simulink model "RedCrane_Merged_control_12032025"  (R2024b)
settings: Solver=VariableStepAuto  StartTime=0.0  StopTime=33  RelTol=1e-4
model workspace (MATLAB code in the model file):
  | %% Geometric properties
  | 
  | %Basic geometry width
  | w0 = 0.07;
  | w1 = w0/4;
  | l_RJ = 0.277; %2.1*w0;
  | r_RJ = 0.030;
  | 
  | %Column geometry
  | L_Column = 1.5655; %2;
  | eta_B = -0.25;
  | zeta_B = L_Column;
  | eta_D = -0.365; %0.25;
  | zeta_D = 1.4805; %1.5;
  | eta_J = 0.200; % 0.25;
  | zeta_J = 0.1195; %0.25;
  | 
  | %Column - Main boom link
  | l_DE = 0.490; % 0.5;
  | l_FE = 0.170; % 0.4;
  | 
  | %Main boom geometry
  | L_Mboom = 2.400; % 2;
  | eta_C = 2.400; % 2;
  | zeta_C = 0.070; % 0.25;
  | eta_F = 0.340; % 0.6;
  | zeta_F = 0.010; % -0.25;
  | eta_G = 2.365; % 1.75;
  | zeta_G = 0.235; % -0.25;
  | eta_K = 0.750; % 1;
  | zeta_K = 0.045; % -0.25;
  | 
  | %Main boom-Jib boom link
  | l_GH = 0.490; % 0.5;
  | l_IH = 0.220; % 0.4;
  | 
  | %Jib boom geometry
  | L_Jib_boom = 2.429; % 2;
  | eta_I = 0.280; % 0.5;
  | zeta_I = 0.005; % -0.25;
  | eta_TP = L_Jib_boom;
  | zeta_TP = 0;
  | 
  | % Winch
  | r_W = 0.205/2;
  | L_W = 0.191;
  | eta_W = 0.28722;
  | zeta_W = -0.29926;
  | beta_W = -0.335;
  | 
  | % Mounting plate
  | eta_MP = -0.0249;
  | zeta_MP = -0.17479;
  | beta_MP = 0;
  | 
  | % Pulley
  | r_P = 0.210/2; % Radius pulley
  | eta_P = 2.140;
  | zeta_P = -0.0506;
  | beta_P = -0.0;
  | 
  | %Roller
  | r_RO = 0.055/2; % Radius roller over
  | r_RU = 0.046/2; % Radius roller under
  | eta_RO = 0.306;
  | zeta_RO = 0.12510;
  | 
  | %Mounting
  | L_M = 1; %m
  | W_M = 1; %m
  | H_M = 1; %m
  | eta_M = 0; %m
  | zeta_M = -0.5; %m
  | beta_M = 0; %m
  | 
  | %Ground
  | L_ground = 6; %m
  | W_ground = 4; %m
  | H_ground = 0.01; %m
  | eta_ground = 1.5; %m
  | zeta_ground = -0.5; %m
  | beta_ground = 0; %m
  | 
  | 
  | %% Mass properties (Mass and center of mass)
  | column_mass = 239.4; % kg
  | column_COM = [-0.1007, 0.0001, 0.4351]; % m
  | 
  | MainBoom_mass = 216.5; % kg
  | MainBoom_COM = [1.134, 0.1674, -0.0018]; % m
  | 
  | JibBoom_mass = 842.2; % kg
  | JibBoom_COM = [0.9806, 0.1814, -0.2939]; % m
  | 
  | % Dogbone
  | E2F_mass = 7.076*2; % kg
  | E2F_COM = [0.0817, 0, 0]; % m
  | 
  | D2E_mass = 6.426*2; % kg
  | D2E_COM = [0.245, 0, 0]; % m
  | 
  | G2H_mass = 6.426*2; % kg
  | G2H_COM = [0.245, 0, 0]; % m
  | 
  | H2I_mass = 22.05; % kg
  | H2I_COM = [0.1206, 0, 0]; % m
  | 
  | % Main cylinder
  | MainC_bottom_mass = 57.9561; % kg
  | MainC_bottom_COM = [0.0081, -0.001, 0.4125]; % m
  | 
  | MainC_rod_mass = 43.93; % kg
  | MainC_rod_COM = [0, 0, -0.4290]; % m
  | 
  | % Jib cylinder
  | JibC_bottom_mass = 55.7738; % kg
  | JibC_bottom_COM = [0.0038, 0.0022, 0.4468]; % m
  | 
  | JibC_rod_mass = 45.8854; % kg
  | JibC_rod_COM = [0, 0, -0.4694]; % m
  | 
  | % Winch
  | Winch_mass = 54; % kg
  | Winch_COM = [0, 0, 0]; % m
  | 
  | 
  | %% Inertia properties (Moments of inertia and products of inertia)
  | 
  | column_MOI = [109, 114, 9.009]; % kg*m^2
  | column_POI = [0.0319, -21.59, -0.0113]; % kg*m^2
  | 
  | MainBoom_MOI = [6.5, 160.3, 160]; % kg*m^2
  | MainBoom_POI = [0.0666, 0.1093, 8.016]; % kg*m^2
  | 
  | JibBoom_MOI = [31.75, 566.3, 573.1]; % kg*m^2
  | JibBoom_POI = [-0.0237, -11.42, 9.588]; % kg*m^2
  | 
  | % Dogbone
  | E2F_MOI = [0.0111, 0.0546, 0.0587]; % kg*m^2
  | E2F_POI = [0, -0.0089, 0]; % kg*m^2
  | 
  | D2E_MOI = [0.0069, 0.2419, 0.2485]; % kg*m^2
  | D2E_POI = [0, 0, 0]; % kg*m^2
  | 
  | G2H_MOI = [0.0069, 0.2419, 0.2485]; % kg*m^2
  | G2H_POI = [0, 0, 0]; % kg*m^2
  | 
  | H2I_MOI = [0.2636, 0.4184, 0.1901]; % kg*m^2
  | H2I_POI = [0, 0, 0]; % kg*m^2
  | 
  | 
  | % Main cylinder
  | MainC_bottom_MOI = [7.2059, 7.2304, 0.3979]; % kg*m^2
  | MainC_bottom_POI = [-0.0126, -0.1802, 0.0002]; % kg*m^2
  | 
  | MainC_rod_MOI = [6.0014, 5.9633, 0.1401]; % kg*m^2
  | MainC_rod_POI = [0, -0.0001, 0]; % kg*m^2
  | 
  | % Jib cylinder
  | JibC_bottom_MOI = [8.3780, 8.3476, 0.3607]; % kg*m^2
  | JibC_bottom_POI = [-0.0119, -0.1037, 0.0033]; % kg*m^2
  | 
  | JibC_rod_MOI = [7.4245, 7.3864, 0.1401]; % kg*m^2
  | JibC_rod_POI = [0, -0.0001, 0]; % kg*m^2
  | 
  | % Winch
  | I_W_xx = (1/4)*Winch_mass*r_W^2 + (1/12)*Winch_mass*L_W^2;
  | I_W_yy = (1/4)*Winch_mass*r_W^2 + (1/12)*Winch_mass*L_W^2;
  | I_W_zz = (1/2)*Winch_mass*r_W^2;
  | 
  | Winch_MOI = [I_W_xx, I_W_yy, I_W_zz]; % kg*m^2
  | Winch_POI = [0, 0, 0]; % kg*m^2
  | 
  | 
  | %% Hydraulics
  | 
  | %-------------Cylinder---------------------
  | 
  | % Main cylinder
  | D_piston_MainC = 160; %mm dimater of piston side
  | L_piston_MainC = 65; %66.2;%mm length from joint to buttom of piston side
  | D_rod_MainC = 100; %mm diamter of cylinder rod
  | L_rod_MainC = 978; %990;%mm length from bottom of rod to joint
  | A_piston_MainC = pi/4*D_piston_MainC^2; % mm^2 area of piston side
  | A_rod_MainC = pi/4*D_rod_MainC^2; % mm^2 area of rod
  | A_rodside_MainC = A_piston_MainC-A_rod_MainC; % mm^2 area of rod side
  | L_barrel_MainC = 945-L_piston_MainC; %mm
  | stroke_MainC = 0.75; %m
  | initial_pos_Main = 0.18; %m
  | initial_Pa_Main = 17;%Bar
  | 
  | % Jib cylinder
  | D_piston_JibC = 150; %mm dimater of piston side
  | L_piston_JibC = 65; %66.2;%mm length from joint to buttom of piston side
  | D_rod_JibC = 100; %mm diamter of cylinder rod
  | L_rod_JibC = 1089.5; %1105.5;%mm length from bottom of rod to joint
  | A_piston_JibC = pi/4*D_piston_JibC^2; % mm^2 area of piston side
  | A_rod_JibC = pi/4*D_rod_JibC^2; % mm^2 area of rod
  | A_rodside_JibC = A_piston_JibC-A_rod_JibC; % mm^2 area of rod side
  | L_barrel_JibC = 1050-L_piston_JibC; %mm
  | stroke_JibC = 0.855; %m
  | initial_pos_Jib = 0.855; %m
  | initial_Pa_Jib = 1;%Bar
  | initial_Pb_Jib = 67;%Bar
  | 
  | % winch
  | poly_b = [1.762740809095876e+02,-44.442169999547330];
  | poly_c = [1.901177983521692e+02,-1.484122102902541e+02];
  | angle_b = poly_b(1)*initial_pos_Main + poly_b(2);
  | angle_c = poly_c(1)*initial_pos_Jib + poly_c(2);
  | angle_w = -90 - angle_c - angle_b;
  | 
  | %Motor
  | DM = 200; %Displacement cm^3/rev
  | GR = 5.04; % Gear ratio 1:5,04
  | 
  | 
  | % ------------------CBV-------------------
  | 
  | % Main
  | pCr_Main = 43.95;%Bar
  | dp_open_Main = 124.43;%Bar
  | 
  | % Jib
  | alpha = 2.7;
  | pCr_Jib_A = 320;%Bar
  | dp_open_Jib_A = 65;%Bar
  | pCr_Jib_B = 280;%Bar
  | dp_open_Jib_B = 40;%Bar
  | 
  | %-------------------DCV-----------------------
  | Cd = 0.64;
  | Q_rat = 30/6e4;
  | dp_2 = 6e5;
  | dp_1 = 1e5;
  | roh = 850;
  | 
  | % Main dcv
  | dead_up_Main = 0.071;
  | dead_down_Main = 0.126;
  | 
  | % Jib dcv
  | dead_up_Jib = 0.037;
  | dead_down_Jib = 0.126;
  | 
  | Ad2 = Q_rat/(Cd*sqrt(2/roh*dp_2))*1e6; %mm
  | Ad1_1 = Q_rat/(Cd*sqrt(2/roh*dp_1))*1e6;
  | Ad1_0 = Q_rat/(Cd*sqrt(2/roh*dp_1))*1e6*0;
  | 
  | Ad1_Main_up = Q_rat/(Cd*sqrt(2/roh*dp_1))*1e6*dead_up_Main;
  | Ad1_Main_down = Q_rat/(Cd*sqrt(2/roh*dp_1))*1e6*dead_down_Main;
  | Ad1_Jib_up = Q_rat/(Cd*sqrt(2/roh*dp_1))*1e6*dead_up_Jib;
  | Ad1_Jib_down = Q_rat/(Cd*sqrt(2/roh*dp_1))*1e6*dead_down_Jib;
undefined symbols (not defined in the file or in its folder): dead_down_m, dead_up_m, X, Y, Z
libraries: sm_lib x171, fl_lib x94, nesl_utility x64, SimscapeFluids_lib x33, sdl_lib x1
(part 4 of 9)

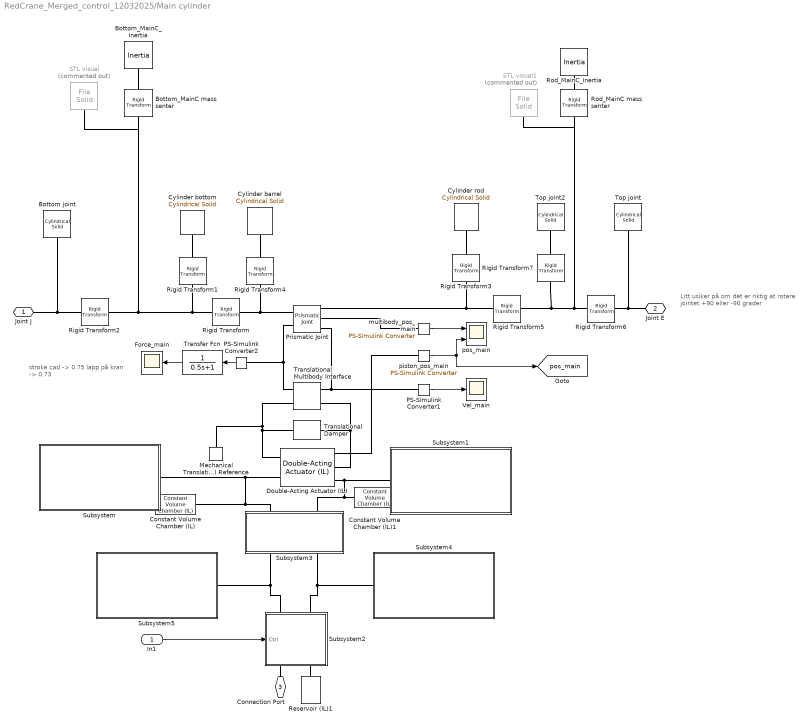
== system RedCrane_Merged_control_12032025/Main cylinder ==
  note: stroke
      | cad -> 0.75
      | lapp på kran -> 0.73
  note: Litt usiker på om det er riktig
      | at rotere jointet +90 eller -90
      | grader
  In1 : Inport
  Bottom joint : sm_lib/Body Elements/Cylindrical Solid  CylinderRadius=0.05  CylinderRadiusUnits=m  CylinderLength=0.2  CylinderLengthUnits=m  ExportEntireGeometry=off  InertiaType=Custom  BasedOnType=Density  Density=1000  DensityUnits=kg/m^3  Mass=0  MassUnits=kg  CenterOfMass=[0 0 0]  CenterOfMassUnits=m  MomentsOfInertia=[0 0 0]  MomentsOfInertiaUnits=kg*m^2  ProductsOfInertia=[0 0 0]  ProductsOfInertiaUnits=kg*m^2  GraphicType=FromGeometry  MarkerShape=Sphere  MarkerSize=10  GraphicVisPropType=SimpleVisualProperties  GraphicDiffuseColor=[0 1 0]  GraphicOpacity=1  GraphicSpecularColor=[0.5 0.5 0.5 1.0]  GraphicAmbientColor=[0.15 0.15 0.15 1.0]  GraphicEmissiveColor=[0.0 0.0 0.0 1.0]  GraphicShininess=75  DoExposeReferenceFrame=on  SerializedFrames=<Frames/>
  Bottom_MainC mass senter : sm_lib/Frames and Transforms/Rigid Transform  RotationMethod=None  FollAlignAxisA=+X  BaseAlignAxisA=+Y  FollAlignAxisB=+Y  BaseAlignAxisB=+Z  RotationStandardAxis=+Z  RotationAngle=0  RotationAngleUnits=deg  RotationArbitraryAxis=[0 0 1]  RotationSequenceAxes=FollowerAxes  RotationSequence=XYX  RotationSequenceAngles=[0 0 0]  RotationSequenceAnglesUnits=deg  RotationMatrix=[1 0 0;0 1 0;0 0 1]  Quaternion=[1 0 0 0]  TranslationMethod=Cartesian  TranslationCartesianOffset=MainC_bottom_COM  TranslationCartesianOffsetUnits=m  TranslationStandardAxis=+Z  TranslationStandardOffset=0  TranslationStandardOffsetUnits=m  TranslationROffset=0  TranslationROffsetUnits=m  TranslationThetaOffset=0  TranslationThetaOffsetUnits=deg  TranslationZOffset=0  TranslationZOffsetUnits=m
  Bottom_MainC_Inertia : sm_lib/Body Elements/Inertia  InertiaType=Custom  Mass=MainC_bottom_mass  MassUnits=kg  CenterOfMass=[0,0,0]  CenterOfMassUnits=m  MomentsOfInertia=MainC_bottom_MOI  MomentsOfInertiaUnits=kg*m^2  ProductsOfInertia=MainC_bottom_POI  ProductsOfInertiaUnits=kg*m^2  GraphicType=Marker  MarkerShape=Sphere  MarkerSize=20  GraphicVisPropType=SimpleVisualProperties  GraphicDiffuseColor=[1 0 1]  GraphicOpacity=1  GraphicSpecularColor=[0.5 0.5 0.5 1.0]  GraphicAmbientColor=[0.15 0.15 0.15 1.0]  GraphicEmissiveColor=[0.0 0.0 0.0 1.0]  GraphicShininess=75
  Constant Volume Chamber (IL) : fl_lib/Isothermal Liquid/Elements/Constant Volume Chamber (IL)  volume=0.001 m^3  p_I_specify=on  p_I_priority=High  p_I=initial_Pa_Main bar  p_I_nominal_specify=off  p_I_nominal_value=1  p_I_nominal_unit=MPa
      settings: InternalSimscapePortConfiguration="{\"Bottom\":[],\"Left\":[{\"id\":\"A\",\"label\":\"A\",\"type\":\"foundation.isothermal_liquid.isothermal_liquid\"}],\"Right\":[],\"Top\":[]}"
  Constant Volume Chamber (IL)1 : fl_lib/Isothermal Liquid/Elements/Constant Volume Chamber (IL)  volume=0.001 m^3  p_I_specify=on  p_I_priority=High  p_I=47 bar  p_I_nominal_specify=off  p_I_nominal_value=1  p_I_nominal_unit=MPa
      settings: InternalSimscapePortConfiguration="{\"Bottom\":[],\"Left\":[{\"id\":\"A\",\"label\":\"A\",\"type\":\"foundation.isothermal_liquid.isothermal_liquid\"}],\"Right\":[],\"Top\":[]}"
  Cylinder barrel : sm_lib/Body Elements/Cylindrical Solid  CylinderRadius=D_piston_MainC/2  CylinderRadiusUnits=mm  CylinderLength=L_barrel_MainC  CylinderLengthUnits=mm  ExportEntireGeometry=off  InertiaType=Custom  BasedOnType=Density  Density=1000  DensityUnits=kg/m^3  Mass=0  MassUnits=kg  CenterOfMass=[0 0 0]  CenterOfMassUnits=m  MomentsOfInertia=[0 0 0]  MomentsOfInertiaUnits=kg*m^2  ProductsOfInertia=[0 0 0]  ProductsOfInertiaUnits=kg*m^2  GraphicType=FromGeometry  MarkerShape=Sphere  MarkerSize=10  GraphicVisPropType=SimpleVisualProperties  GraphicDiffuseColor=[0 1 0]  GraphicOpacity=1  GraphicSpecularColor=[0.5 0.5 0.5 1.0]  GraphicAmbientColor=[0.15 0.15 0.15 1.0]  GraphicEmissiveColor=[0.0 0.0 0.0 1.0]  GraphicShininess=75  DoExposeReferenceFrame=on  SerializedFrames=<Frames/>
  Cylinder bottom : sm_lib/Body Elements/Cylindrical Solid  CylinderRadius=D_piston_MainC/2  CylinderRadiusUnits=mm  CylinderLength=L_piston_MainC  CylinderLengthUnits=mm  ExportEntireGeometry=off  InertiaType=Custom  BasedOnType=Density  Density=1000  DensityUnits=kg/m^3  Mass=0.001  MassUnits=g  CenterOfMass=[0 0 0]  CenterOfMassUnits=m  MomentsOfInertia=[1 1 1]  MomentsOfInertiaUnits=kg*m^2  ProductsOfInertia=[0 0 0]  ProductsOfInertiaUnits=kg*m^2  GraphicType=FromGeometry  MarkerShape=Sphere  MarkerSize=10  GraphicVisPropType=SimpleVisualProperties  GraphicDiffuseColor=[0 1 0]  GraphicOpacity=1  GraphicSpecularColor=[0.5 0.5 0.5 1.0]  GraphicAmbientColor=[0.15 0.15 0.15 1.0]  GraphicEmissiveColor=[0.0 0.0 0.0 1.0]  GraphicShininess=75  DoExposeReferenceFrame=on  SerializedFrames=<Frames/>
  Cylinder rod : sm_lib/Body Elements/Cylindrical Solid  CylinderRadius=D_rod_MainC/2  CylinderRadiusUnits=mm  CylinderLength=L_rod_MainC  CylinderLengthUnits=mm  ExportEntireGeometry=off  InertiaType=Custom  BasedOnType=Density  Density=1000  DensityUnits=kg/m^3  Mass=0.001  MassUnits=g  CenterOfMass=[0 0 0]  CenterOfMassUnits=m  MomentsOfInertia=[0 0 0]  MomentsOfInertiaUnits=kg*m^2  ProductsOfInertia=[0 0 0]  ProductsOfInertiaUnits=kg*m^2  GraphicType=FromGeometry  MarkerShape=Sphere  MarkerSize=10  GraphicVisPropType=SimpleVisualProperties  GraphicDiffuseColor=[0 0 1]  GraphicOpacity=1  GraphicSpecularColor=[0.5 0.5 0.5 1.0]  GraphicAmbientColor=[0.15 0.15 0.15 1.0]  GraphicEmissiveColor=[0.0 0.0 0.0 1.0]  GraphicShininess=75  DoExposeReferenceFrame=on  SerializedFrames=<Frames/>
  Double-Acting Actuator (IL) : SimscapeFluids_lib/Isothermal Liquid/Actuators/Double-Acting Actuator (IL)  single_fluid=true  mech_orientation=foundation.enum.MechOrientationTranslational.Positive  piston_area_A=A_piston_MainC mm^2  piston_area_B=A_rodside_MainC mm^2  stroke=stroke_MainC m  dead_volume_A=1e-5 m^3  dead_volume_B=1e-5 m^3  pressure_spec=foundation.enum.pressure_spec.atmospheric  environment_pressure=0.101325 MPa  hardstop_model=simscape.enum.hardstop.smooth  stiff_coeff=1e10 N/m  damping_coeff=150 N*s/m  transition=0.1 mm  coeff_rest=0.7  v_tol=0.001 m/s  f_tol=0.001 N  cushion_A_spec=false  area_plunger_A=1e-4 m^2  length_plunger_A=1e-3 m  area_cushion_orifice_A=1e-6 m^2  area_leak_plunger_A=1e-7 m^2  p_crack_differential_A=0.01 MPa  press_max_differential_A=0.1 MPa  check_valve_area_max_A=1e-4 m^2  check_valve_area_leak_A=1e-10 m^2  smoothing_factor_A=0.01  cushion_B_spec=false  area_plunger_B=1e-4 m^2  length_plunger_B=1e-3 m  area_cushion_orifice_B=1e-6 m^2  area_leak_plunger_B=1e-7 m^2  p_crack_differential_B=0.01 MPa  press_max_differential_B=0.1 MPa  check_valve_area_max_B=1e-4 m^2  check_valve_area_leak_B=1e-10 m^2  smoothing_factor_B=0.01  friction_spec=true  breakaway_Coulomb_ratio=1.2  breakaway_velocity=0.1 m/s  preload_force=20 N  Coulomb_coeff=20e-6 N/Pa  viscous_coeff=100 N*s/m  leakage_spec=false  clearance=1e-4 m  piston_length=0.01 m  displacement_spec=foundation.enum.DisplacementSpec.Calculate  x0=initial_pos_Main m  dynamic_compressibility=true  p0_A=initial_Pa_Main bar  p0_B=1 bar
      settings: InternalSimscapePortConfiguration="{\"Bottom\":[],\"Left\":[{\"id\":\"C\",\"label\":\"C\",\"type\":\"foundation.mechanical.translational.translational\"},{\"id\":\"A\",\"label\":\"A\",\"type\":\"foundation.isothermal_liquid.isothermal_liquid\"}],\"Right\":[{\"id\":\"p_out\",\"label\":\"p\",\"type\":\"output\"},{\"id\":\"R\",\"label\":\"R\",\"type\":\"foundation.mechanical.translational.translational\"},{\"id\":\"B\",\"label\":\"B\",\"type\":\"foundation.isothermal_liquid.isothermal_liquid\"}],\"Top\":[]}"
  Force_main : Scope
  Mechanical Translational Reference : fl_lib/Mechanical/Translational Elements/Mechanical Translational Reference
  PS-Simulink Converter1 : nesl_utility/PS-Simulink Converter  PhysicalDomain=network_engine_domain  SubClassName=ps_output  LeftPortType=input  RightPortType=output  PseudoPeriodic=off  Frequencies=[]  VectorFormat=inherit  Unit=inherit  AffineConversion=off
  PS-Simulink Converter2 : nesl_utility/PS-Simulink Converter  PhysicalDomain=network_engine_domain  SubClassName=ps_output  LeftPortType=input  RightPortType=output  PseudoPeriodic=off  Frequencies=[]  VectorFormat=inherit  Unit=inherit  AffineConversion=off
  Prismatic Joint : sm_lib/Joints/Prismatic Joint  JointMode=Normal  CompositeWrenchDir=FollowerOnBase  CompositeWrenchFrame=BaseFrame  SenseConstraintForce=off  SenseConstraintTorque=off  SenseTotalForce=off  SenseTotalTorque=off  PositionTargetSpecify=on  PositionTargetPriority=High  PositionTargetValue=initial_pos_Main  PositionTargetValueUnits=m  VelocityTargetSpecify=off  VelocityTargetPriority=High  VelocityTargetValue=0  VelocityTargetValueUnits=m/s  EquilibriumPosition=0  EquilibriumPositionUnits=m  SpringStiffness=0  SpringStiffnessUnits=N/m  DampingCoefficient=0  DampingCoefficientUnits=N/(m/s)  LowerLimitSpecify=off  LowerLimitBound=0  LowerLimitBoundUnits=m  LowerLimitStiffness=1e6  LowerLimitStiffnessUnits=N/m  LowerLimitDamping=1e3  LowerLimitDampingUnits=N/(m/s)  LowerLimitTransitionRegionWidth=1e-4  LowerLimitTransitionRegionWidthUnits=m  UpperLimitSpecify=off  UpperLimitBound=stroke_MainC  UpperLimitBoundUnits=m  UpperLimitStiffness=1e6  UpperLimitStiffnessUnits=N/m  UpperLimitDamping=1e3  UpperLimitDampingUnits=N/(m/s)  UpperLimitTransitionRegionWidth=1e-4  UpperLimitTransitionRegionWidthUnits=m  TorqueActuationMode=InputTorque  MotionActuationMode=ComputedMotion  SensePosition=on  SenseVelocity=on  SenseAcceleration=off  SenseTorqueForce=off  SenseLowerLimitTorqueForce=off  SenseUpperLimitTorqueForce=off
  Reservoir (IL)1 : fl_lib/Isothermal Liquid/Elements/Reservoir (IL)  reservoir_type=foundation.enum.constant_controlled.constant  pressure_spec=foundation.enum.pressure_spec.atmospheric  reservoir_pressure=0.101325 MPa
  Rigid Transform : sm_lib/Frames and Transforms/Rigid Transform  RotationMethod=None  FollAlignAxisA=+X  BaseAlignAxisA=+Y  FollAlignAxisB=+Y  BaseAlignAxisB=+Z  RotationStandardAxis=+Z  RotationAngle=0  RotationAngleUnits=deg  RotationArbitraryAxis=[0 0 1]  RotationSequenceAxes=FollowerAxes  RotationSequence=XYX  RotationSequenceAngles=[0 0 0]  RotationSequenceAnglesUnits=deg  RotationMatrix=[1 0 0;0 1 0;0 0 1]  Quaternion=[1 0 0 0]  TranslationMethod=Cartesian  TranslationCartesianOffset=[0 0 L_piston_JibC]  TranslationCartesianOffsetUnits=mm  TranslationStandardAxis=+Z  TranslationStandardOffset=0  TranslationStandardOffsetUnits=m  TranslationROffset=0  TranslationROffsetUnits=m  TranslationThetaOffset=0  TranslationThetaOffsetUnits=deg  TranslationZOffset=0  TranslationZOffsetUnits=m
  Rigid Transform1 : sm_lib/Frames and Transforms/Rigid Transform  RotationMethod=None  FollAlignAxisA=+X  BaseAlignAxisA=+Y  FollAlignAxisB=+Y  BaseAlignAxisB=+Z  RotationStandardAxis=+Z  RotationAngle=0  RotationAngleUnits=deg  RotationArbitraryAxis=[0 0 1]  RotationSequenceAxes=FollowerAxes  RotationSequence=XYX  RotationSequenceAngles=[0 0 0]  RotationSequenceAnglesUnits=deg  RotationMatrix=[1 0 0;0 1 0;0 0 1]  Quaternion=[1 0 0 0]  TranslationMethod=Cartesian  TranslationCartesianOffset=[0 0 L_piston_MainC/2]  TranslationCartesianOffsetUnits=mm  TranslationStandardAxis=+Z  TranslationStandardOffset=0  TranslationStandardOffsetUnits=m  TranslationROffset=0  TranslationROffsetUnits=m  TranslationThetaOffset=0  TranslationThetaOffsetUnits=deg  TranslationZOffset=0  TranslationZOffsetUnits=m
  Rigid Transform2 : sm_lib/Frames and Transforms/Rigid Transform  RotationMethod=StandardAxis  FollAlignAxisA=+X  BaseAlignAxisA=+Y  FollAlignAxisB=+Y  BaseAlignAxisB=+Z  RotationStandardAxis=+X  RotationAngle=-90  RotationAngleUnits=deg  RotationArbitraryAxis=[0 0 1]  RotationSequenceAxes=FollowerAxes  RotationSequence=XYX  RotationSequenceAngles=[0 0 0]  RotationSequenceAnglesUnits=deg  RotationMatrix=[1 0 0;0 1 0;0 0 1]  Quaternion=[1 0 0 0]  TranslationMethod=None  TranslationCartesianOffset=[0 0 0]  TranslationCartesianOffsetUnits=m  TranslationStandardAxis=+Z  TranslationStandardOffset=0  TranslationStandardOffsetUnits=m  TranslationROffset=0  TranslationROffsetUnits=m  TranslationThetaOffset=0  TranslationThetaOffsetUnits=deg  TranslationZOffset=0  TranslationZOffsetUnits=m
  Rigid Transform3 : sm_lib/Frames and Transforms/Rigid Transform  RotationMethod=None  FollAlignAxisA=+X  BaseAlignAxisA=+Y  FollAlignAxisB=+Y  BaseAlignAxisB=+Z  RotationStandardAxis=+Z  RotationAngle=0  RotationAngleUnits=deg  RotationArbitraryAxis=[0 0 1]  RotationSequenceAxes=FollowerAxes  RotationSequence=XYX  RotationSequenceAngles=[0 0 0]  RotationSequenceAnglesUnits=deg  RotationMatrix=[1 0 0;0 1 0;0 0 1]  Quaternion=[1 0 0 0]  TranslationMethod=Cartesian  TranslationCartesianOffset=[0 0 L_rod_MainC/2]  TranslationCartesianOffsetUnits=mm  TranslationStandardAxis=+Z  TranslationStandardOffset=0  TranslationStandardOffsetUnits=m  TranslationROffset=0  TranslationROffsetUnits=m  TranslationThetaOffset=0  TranslationThetaOffsetUnits=deg  TranslationZOffset=0  TranslationZOffsetUnits=m
  Rigid Transform4 : sm_lib/Frames and Transforms/Rigid Transform  RotationMethod=None  FollAlignAxisA=+X  BaseAlignAxisA=+Y  FollAlignAxisB=+Y  BaseAlignAxisB=+Z  RotationStandardAxis=+Z  RotationAngle=0  RotationAngleUnits=deg  RotationArbitraryAxis=[0 0 1]  RotationSequenceAxes=FollowerAxes  RotationSequence=XYX  RotationSequenceAngles=[0 0 0]  RotationSequenceAnglesUnits=deg  RotationMatrix=[1 0 0;0 1 0;0 0 1]  Quaternion=[1 0 0 0]  TranslationMethod=Cartesian  TranslationCartesianOffset=[0 0 L_barrel_MainC/2]  TranslationCartesianOffsetUnits=mm  TranslationStandardAxis=+Z  TranslationStandardOffset=0  TranslationStandardOffsetUnits=m  TranslationROffset=0  TranslationROffsetUnits=m  TranslationThetaOffset=0  TranslationThetaOffsetUnits=deg  TranslationZOffset=0  TranslationZOffsetUnits=m
  Rigid Transform5 : sm_lib/Frames and Transforms/Rigid Transform  RotationMethod=None  FollAlignAxisA=+X  BaseAlignAxisA=+Y  FollAlignAxisB=+Y  BaseAlignAxisB=+Z  RotationStandardAxis=+Z  RotationAngle=0  RotationAngleUnits=deg  RotationArbitraryAxis=[0 0 1]  RotationSequenceAxes=FollowerAxes  RotationSequence=XYX  RotationSequenceAngles=[0 0 0]  RotationSequenceAnglesUnits=deg  RotationMatrix=[1 0 0;0 1 0;0 0 1]  Quaternion=[1 0 0 0]  TranslationMethod=Cartesian  TranslationCartesianOffset=[0 0 L_rod_MainC]  TranslationCartesianOffsetUnits=mm  TranslationStandardAxis=+Z  TranslationStandardOffset=0  TranslationStandardOffsetUnits=m  TranslationROffset=0  TranslationROffsetUnits=m  TranslationThetaOffset=0  TranslationThetaOffsetUnits=deg  TranslationZOffset=0  TranslationZOffsetUnits=m
  Rigid Transform6 : sm_lib/Frames and Transforms/Rigid Transform  RotationMethod=StandardAxis  FollAlignAxisA=+X  BaseAlignAxisA=+Y  FollAlignAxisB=+Y  BaseAlignAxisB=+Z  RotationStandardAxis=+X  RotationAngle=90  RotationAngleUnits=deg  RotationArbitraryAxis=[0 0 1]  RotationSequenceAxes=FollowerAxes  RotationSequence=XYX  RotationSequenceAngles=[0 0 0]  RotationSequenceAnglesUnits=deg  RotationMatrix=[1 0 0;0 1 0;0 0 1]  Quaternion=[1 0 0 0]  TranslationMethod=None  TranslationCartesianOffset=[0 0 0]  TranslationCartesianOffsetUnits=m  TranslationStandardAxis=+Z  TranslationStandardOffset=0  TranslationStandardOffsetUnits=m  TranslationROffset=0  TranslationROffsetUnits=m  TranslationThetaOffset=0  TranslationThetaOffsetUnits=deg  TranslationZOffset=0  TranslationZOffsetUnits=m
  Rigid Transform7 : sm_lib/Frames and Transforms/Rigid Transform  RotationMethod=None  FollAlignAxisA=+X  BaseAlignAxisA=+Y  FollAlignAxisB=+Y  BaseAlignAxisB=+Z  RotationStandardAxis=+Z  RotationAngle=0  RotationAngleUnits=deg  RotationArbitraryAxis=[0 0 1]  RotationSequenceAxes=FollowerAxes  RotationSequence=XYX  RotationSequenceAngles=[0 0 0]  RotationSequenceAnglesUnits=deg  RotationMatrix=[1 0 0;0 1 0;0 0 1]  Quaternion=[1 0 0 0]  TranslationMethod=Cartesian  TranslationCartesianOffset=[0 0 -75]  TranslationCartesianOffsetUnits=mm  TranslationStandardAxis=+Z  TranslationStandardOffset=0  TranslationStandardOffsetUnits=m  TranslationROffset=0  TranslationROffsetUnits=m  TranslationThetaOffset=0  TranslationThetaOffsetUnits=deg  TranslationZOffset=0  TranslationZOffsetUnits=m
  Rod_MainC mass senter : sm_lib/Frames and Transforms/Rigid Transform  RotationMethod=None  FollAlignAxisA=+X  BaseAlignAxisA=+Y  FollAlignAxisB=+Y  BaseAlignAxisB=+Z  RotationStandardAxis=+Z  RotationAngle=0  RotationAngleUnits=deg  RotationArbitraryAxis=[0 0 1]  RotationSequenceAxes=FollowerAxes  RotationSequence=XYX  RotationSequenceAngles=[0 0 0]  RotationSequenceAnglesUnits=deg  RotationMatrix=[1 0 0;0 1 0;0 0 1]  Quaternion=[1 0 0 0]  TranslationMethod=Cartesian  TranslationCartesianOffset=MainC_rod_COM  TranslationCartesianOffsetUnits=m  TranslationStandardAxis=+Z  TranslationStandardOffset=0  TranslationStandardOffsetUnits=m  TranslationROffset=0  TranslationROffsetUnits=m  TranslationThetaOffset=0  TranslationThetaOffsetUnits=deg  TranslationZOffset=0  TranslationZOffsetUnits=m
  Rod_MainC_Inertia : sm_lib/Body Elements/Inertia  InertiaType=Custom  Mass=MainC_rod_mass  MassUnits=kg  CenterOfMass=[0,0,0]  CenterOfMassUnits=m  MomentsOfInertia=MainC_rod_MOI  MomentsOfInertiaUnits=kg*m^2  ProductsOfInertia=MainC_rod_POI  ProductsOfInertiaUnits=kg*m^2  GraphicType=Marker  MarkerShape=Sphere  MarkerSize=20  GraphicVisPropType=SimpleVisualProperties  GraphicDiffuseColor=[1 0 1]  GraphicOpacity=1  GraphicSpecularColor=[0.5 0.5 0.5 1.0]  GraphicAmbientColor=[0.15 0.15 0.15 1.0]  GraphicEmissiveColor=[0.0 0.0 0.0 1.0]  GraphicShininess=75
  STL visual : sm_lib/Body Elements/File Solid  Commented=on  ExtGeomFileName=pully.STL  UnitType=Custom  ExtGeomFileUnits=mm  StepReaderType=HEX  ExportConvexHullGeometry=off  InertiaType=Custom  BasedOnType=DensityFromFile  Density=1000  DensityUnits=kg/m^3  Mass=0  MassUnits=kg  CenterOfMass=[0 0 0]  CenterOfMassUnits=m  MomentsOfInertia=[0 0 0]  MomentsOfInertiaUnits=kg*m^2  ProductsOfInertia=[0 0 0]  ProductsOfInertiaUnits=kg*m^2  GraphicType=FromGeometry  MarkerShape=Sphere  MarkerSize=10  GraphicVisPropType=SimpleVisualProperties  GraphicDiffuseColor=[0.502 0.502 0.502]  GraphicOpacity=1  GraphicSpecularColor=[0 1 0]  GraphicAmbientColor=[0 0.4471 0.7412]  GraphicEmissiveColor=[0.05882 1 1]  GraphicShininess=75  DoExposeReferenceFrame=on  SerializedFrames=<Frames/>
  STL visual1 : sm_lib/Body Elements/File Solid  Commented=on  ExtGeomFileName=pully.STL  UnitType=Custom  ExtGeomFileUnits=mm  StepReaderType=HEX  ExportConvexHullGeometry=off  InertiaType=Custom  BasedOnType=DensityFromFile  Density=1000  DensityUnits=kg/m^3  Mass=0  MassUnits=kg  CenterOfMass=[0 0 0]  CenterOfMassUnits=m  MomentsOfInertia=[0 0 0]  MomentsOfInertiaUnits=kg*m^2  ProductsOfInertia=[0 0 0]  ProductsOfInertiaUnits=kg*m^2  GraphicType=FromGeometry  MarkerShape=Sphere  MarkerSize=10  GraphicVisPropType=SimpleVisualProperties  GraphicDiffuseColor=[0.502 0.502 0.502]  GraphicOpacity=1  GraphicSpecularColor=[0 1 0]  GraphicAmbientColor=[0 0.4471 0.7412]  GraphicEmissiveColor=[0.05882 1 1]  GraphicShininess=75  DoExposeReferenceFrame=on  SerializedFrames=<Frames/>
  Subsystem : Subsystem
  Subsystem1 : Subsystem
  Subsystem2 : Subsystem
      settings: PortSchema="{\"entries\":[{\"content\":{\"sides\":[{\"content\":{\"connectorIds\":[\"In1\"]},\"type\":\"ConnectorPlacement.EquallySpacedRectSide\",\"uuid\":\"6993dbde-6cba-46a2-b1d5-f1047b136426\"},{\"content\":{\"side\":\"RIGHT\"},\"type\":\"ConnectorPlacement.EquallySpacedRectSide\",\"uuid\":\"3ad9b2a3-36be-44b7-a33f-fa48c865a093\"},{\"content\":{\"connectorIds\":[\"LConn1\",\"LConn2\"],\"side\":\"TOP\"},\"type\":\"ConnectorPlacement.EquallySpacedRectSide\",\"uuid\":\"66e9811c-0a42-4ab5-bd83-e8b75281c572\"},{\"content\":{\"connectorIds\":[\"RConn1\",\"RConn2\"],\"side\":\"BOTTOM\"},\"type\":\"ConnectorPlacement.EquallySpacedRectSide\",\"uuid\":\"046bb913-9a9e-4ef9-939b-8e65f57c81b5\"}]},\"type\":\"ConnectorPlacement.EquallySpacedConnector\",\"uuid\":\"5e1ffb91-7437-41ca-a8e1-7c47f283d11a\"}],\"packageUris\":[\"http://schema.mathworks.com/mf0/Connector/R2020b\"],\"version\":\"1.0\"}"
  Subsystem3 : Subsystem
      settings: PortSchema="{\"entries\":[{\"content\":{\"sides\":[{\"content\":{},\"type\":\"ConnectorPlacement.EquallySpacedRectSide\",\"uuid\":\"a9f0eaf7-f148-41af-883d-8aedf66e3fe7\"},{\"content\":{\"side\":\"RIGHT\"},\"type\":\"ConnectorPlacement.EquallySpacedRectSide\",\"uuid\":\"b7d06a0e-217c-4594-9653-b1704beb7fcf\"},{\"content\":{\"connectorIds\":[\"LConn1\",\"LConn2\"],\"side\":\"TOP\"},\"type\":\"ConnectorPlacement.EquallySpacedRectSide\",\"uuid\":\"8b0b6e4d-8977-4f79-be82-c14ccdce2671\"},{\"content\":{\"connectorIds\":[\"RConn1\",\"RConn2\"],\"side\":\"BOTTOM\"},\"type\":\"ConnectorPlacement.EquallySpacedRectSide\",\"uuid\":\"d5bd5d30-b17c-4999-a2e1-ca2e0a57ee34\"}]},\"type\":\"ConnectorPlacement.EquallySpacedConnector\",\"uuid\":\"f712f636-cf3b-4e26-b860-5f0ebbe71685\"}],\"packageUris\":[\"http://schema.mathworks.com/mf0/Connector/R2020b\"],\"version\":\"1.0\"}"
  Subsystem4 : Subsystem
  Subsystem5 : Subsystem
  Top joint : sm_lib/Body Elements/Cylindrical Solid  CylinderRadius=0.06  CylinderRadiusUnits=m  CylinderLength=0.2  CylinderLengthUnits=m  ExportEntireGeometry=off  InertiaType=Custom  BasedOnType=Density  Density=1000  DensityUnits=kg/m^3  Mass=0  MassUnits=kg  CenterOfMass=[0 0 0]  CenterOfMassUnits=m  MomentsOfInertia=[0 0 0]  MomentsOfInertiaUnits=kg*m^2  ProductsOfInertia=[0 0 0]  ProductsOfInertiaUnits=kg*m^2  GraphicType=FromGeometry  MarkerShape=Sphere  MarkerSize=10  GraphicVisPropType=SimpleVisualProperties  GraphicDiffuseColor=[0 0 1]  GraphicOpacity=1  GraphicSpecularColor=[0.5 0.5 0.5 1.0]  GraphicAmbientColor=[0.15 0.15 0.15 1.0]  GraphicEmissiveColor=[0.0 0.0 0.0 1.0]  GraphicShininess=75  DoExposeReferenceFrame=on  SerializedFrames=<Frames/>
  Top joint2 : sm_lib/Body Elements/Cylindrical Solid  CylinderRadius=60  CylinderRadiusUnits=mm  CylinderLength=75  CylinderLengthUnits=mm  ExportEntireGeometry=off  InertiaType=Custom  BasedOnType=Density  Density=1000  DensityUnits=kg/m^3  Mass=0  MassUnits=kg  CenterOfMass=[0 0 0]  CenterOfMassUnits=m  MomentsOfInertia=[0 0 0]  MomentsOfInertiaUnits=kg*m^2  ProductsOfInertia=[0 0 0]  ProductsOfInertiaUnits=kg*m^2  GraphicType=FromGeometry  MarkerShape=Sphere  MarkerSize=10  GraphicVisPropType=SimpleVisualProperties  GraphicDiffuseColor=[0 0 1]  GraphicOpacity=1  GraphicSpecularColor=[0.5 0.5 0.5 1.0]  GraphicAmbientColor=[0.15 0.15 0.15 1.0]  GraphicEmissiveColor=[0.0 0.0 0.0 1.0]  GraphicShininess=75  DoExposeReferenceFrame=on  SerializedFrames=<Frames/>
  Transfer Fcn : TransferFcn  Denominator=[0.5 1]
  Translational Multibody Interface : fl_lib/Mechanical/Multibody Interfaces/Translational Multibody Interface
  Translational Damper : fl_lib/Mechanical/Translational Elements/Translational Damper  D=1e6 N*s/m  v_specify=on  v_priority=Low  v=0 m/s  v_nominal_specify=off  v_nominal_value=1  v_nominal_unit=m/s  f_specify=on  f_priority=High  f=8e5 N  f_nominal_specify=off  f_nominal_value=1  f_nominal_unit=N
  Vel_main : Scope
  multibody_pos_main : nesl_utility/PS-Simulink Converter  PhysicalDomain=network_engine_domain  SubClassName=ps_output  LeftPortType=input  RightPortType=output  PseudoPeriodic=off  Frequencies=[]  VectorFormat=inherit  Unit=inherit  AffineConversion=off
  piston_pos_main : nesl_utility/PS-Simulink Converter  PhysicalDomain=network_engine_domain  SubClassName=ps_output  LeftPortType=input  RightPortType=output  PseudoPeriodic=off  Frequencies=[]  VectorFormat=inherit  Unit=inherit  AffineConversion=off
  pos_main : Scope  NumInputPorts=2
  Joint J : PMIOPort  Side=Left
  Joint E : PMIOPort  Port=2  Side=Right
  Connection Port : PMIOPort  Port=3  Side=Right
  tag scope: pos_main=global
  wires:
  multibody_pos_main/1 -> pos_main/1
  PS-Simulink Converter1/1 -> Vel_main/1
  piston_pos_main/1 -> [pos_main], pos_main/2
  In1/1 -> Subsystem2/1(Ctrl)
  Transfer Fcn/1 -> Force_main/1
  PS-Simulink Converter2/1 -> Transfer Fcn/1
  connections:
  Rigid Transform/LConn1 -- STL visual/RConn1 -- Bottom_MainC mass senter/LConn1 -- Rigid Transform2/RConn1 -- Rigid Transform1/LConn1
  Top joint/RConn1 -- Joint E/RConn1 -- Rigid Transform6/RConn1
  Cylinder bottom/RConn1 -- Rigid Transform1/RConn1
  Bottom joint/RConn1 -- Rigid Transform2/LConn1 -- Joint J/RConn1
  Cylinder rod/RConn1 -- Rigid Transform3/RConn1
  Cylinder barrel/RConn1 -- Rigid Transform4/RConn1
  Rigid Transform/RConn1 -- Rigid Transform4/LConn1 -- Prismatic Joint/LConn1
  Rigid Transform5/RConn1 -- Rigid Transform7/LConn1 -- STL visual1/RConn1 -- Rod_MainC mass senter/LConn1 -- Rigid Transform6/LConn1
  Rigid Transform3/LConn1 -- Prismatic Joint/RConn1 -- Rigid Transform5/LConn1
  Rigid Transform7/RConn1 -- Top joint2/RConn1
  multibody_pos_main/LConn1 -- Prismatic Joint/RConn2
  Double-Acting Actuator (IL)/RConn2 -- Translational Damper/LConn1 -- Translational Multibody Interface/RConn2
  Double-Acting Actuator (IL)/LConn1 -- Translational Damper/RConn1 -- Translational Multibody Interface/LConn2 -- Mechanical Translational Reference/LConn1
  Constant Volume Chamber (IL)/LConn1 -- Subsystem3/LConn1 -- Subsystem/RConn1 -- Double-Acting Actuator (IL)/LConn2
  Subsystem1/RConn1 -- Constant Volume Chamber (IL)1/LConn1 -- Subsystem3/LConn2 -- Double-Acting Actuator (IL)/RConn3
  Translational Multibody Interface/LConn1 -- PS-Simulink Converter2/LConn1 -- Prismatic Joint/LConn2
  Prismatic Joint/RConn3 -- PS-Simulink Converter1/LConn1 -- Translational Multibody Interface/RConn1
  Double-Acting Actuator (IL)/RConn1 -- piston_pos_main/LConn1
  Connection Port/RConn1 -- Subsystem2/RConn1
  Reservoir (IL)1/LConn1 -- Subsystem2/RConn2
  Subsystem3/RConn2 -- Subsystem2/LConn2 -- Subsystem4/RConn1
  Subsystem3/RConn1 -- Subsystem5/RConn1 -- Subsystem2/LConn1
  Rod_MainC_Inertia/RConn1 -- Rod_MainC mass senter/RConn1
  Bottom_MainC_Inertia/RConn1 -- Bottom_MainC mass senter/RConn1

== system RedCrane_Merged_control_12032025/Pump ==
  Constant1 : Constant  Value=130
  Gain : Gain  Gain=1e5
  Pressure Source (IL) : fl_lib/Isothermal Liquid/Sources/Pressure Source (IL)  source_type=foundation.enum.constant_controlled.controlled  pressure_differential=100 bar
      settings: InternalSimscapePortConfiguration="{\"Bottom\":[],\"Left\":[{\"id\":\"A\",\"label\":\"A\",\"type\":\"foundation.isothermal_liquid.isothermal_liquid\"},{\"id\":\"P\",\"label\":\"P\",\"type\":\"input\"}],\"Right\":[{\"id\":\"B\",\"label\":\"B\",\"type\":\"foundation.isothermal_liquid.isothermal_liquid\"}],\"Top\":[]}"
  Reservoir (IL) : fl_lib/Isothermal Liquid/Elements/Reservoir (IL)  reservoir_type=foundation.enum.constant_controlled.constant  pressure_spec=foundation.enum.pressure_spec.atmospheric  reservoir_pressure=0.101325 MPa
  Simulink-PS Converter1 : nesl_utility/Simulink-PS Converter  PhysicalDomain=network_engine_domain  SubClassName=ps_input  LeftPortType=input  RightPortType=output  PseudoPeriodic=off  Frequencies=[]  NoiseDistribution=none  NoiseParameters=[]  Unit=1  AffineConversion=off  FilteringAndDerivatives=provide  SimscapeFilterOrder=1  InputFilterTimeConstant=0.001  UdotUserProvided=0
  Conn1 : PMIOPort  Side=Right
  wires:
  Constant1/1 -> Gain/1
  Gain/1 -> Simulink-PS Converter1/1
  connections:
  Reservoir (IL)/LConn1 -- Pressure Source (IL)/LConn1
  Simulink-PS Converter1/RConn1 -- Pressure Source (IL)/LConn2
  Pressure Source (IL)/RConn1 -- Conn1/RConn1

== system RedCrane_Merged_control_12032025/Subsystem ==
  Ground : sm_lib/Body Elements/Brick Solid  BrickDimensions=[L_ground W_ground H_ground]  BrickDimensionsUnits=m  ExportEntireGeometry=off  InertiaType=Custom  BasedOnType=Density  Density=1000  DensityUnits=kg/m^3  Mass=0  MassUnits=kg  CenterOfMass=[0 0 0]  CenterOfMassUnits=m  MomentsOfInertia=[0 0 0]  MomentsOfInertiaUnits=kg*m^2  ProductsOfInertia=[0 0 0]  ProductsOfInertiaUnits=kg*m^2  GraphicType=FromGeometry  MarkerShape=Sphere  MarkerSize=10  GraphicVisPropType=SimpleVisualProperties  GraphicDiffuseColor=[0 0 0]  GraphicOpacity=1  GraphicSpecularColor=[0.5 0.5 0.5 1.0]  GraphicAmbientColor=[0.15 0.15 0.15 1.0]  GraphicEmissiveColor=[0.0 0.0 0.0 1.0]  GraphicShininess=75  DoExposeReferenceFrame=on  SerializedFrames=<Frames/>
  Mounting : sm_lib/Body Elements/Brick Solid  BrickDimensions=[L_M W_M H_M]  BrickDimensionsUnits=m  ExportEntireGeometry=off  InertiaType=Custom  BasedOnType=Density  Density=1000  DensityUnits=kg/m^3  Mass=0  MassUnits=kg  CenterOfMass=[0 0 0]  CenterOfMassUnits=m  MomentsOfInertia=[0 0 0]  MomentsOfInertiaUnits=kg*m^2  ProductsOfInertia=[0 0 0]  ProductsOfInertiaUnits=kg*m^2  GraphicType=FromGeometry  MarkerShape=Sphere  MarkerSize=10  GraphicVisPropType=SimpleVisualProperties  GraphicDiffuseColor=[1 0 0]  GraphicOpacity=1  GraphicSpecularColor=[0.5 0.5 0.5 1.0]  GraphicAmbientColor=[0.15 0.15 0.15 1.0]  GraphicEmissiveColor=[0.0 0.0 0.0 1.0]  GraphicShininess=75  DoExposeReferenceFrame=on  SerializedFrames=<Frames/>
  Rigid Transform : sm_lib/Frames and Transforms/Rigid Transform  RotationMethod=None  FollAlignAxisA=+X  BaseAlignAxisA=+Y  FollAlignAxisB=+Y  BaseAlignAxisB=+Z  RotationStandardAxis=+Z  RotationAngle=0  RotationAngleUnits=deg  RotationArbitraryAxis=[0 0 1]  RotationSequenceAxes=FollowerAxes  RotationSequence=XYX  RotationSequenceAngles=[0 0 0]  RotationSequenceAnglesUnits=deg  RotationMatrix=[1 0 0;0 1 0;0 0 1]  Quaternion=[1 0 0 0]  TranslationMethod=Cartesian  TranslationCartesianOffset=[eta_M beta_M zeta_M]  TranslationCartesianOffsetUnits=m  TranslationStandardAxis=+Z  TranslationStandardOffset=0  TranslationStandardOffsetUnits=m  TranslationROffset=0  TranslationROffsetUnits=m  TranslationThetaOffset=0  TranslationThetaOffsetUnits=deg  TranslationZOffset=0  TranslationZOffsetUnits=m
  Rigid Transform1 : sm_lib/Frames and Transforms/Rigid Transform  RotationMethod=None  FollAlignAxisA=+X  BaseAlignAxisA=+Y  FollAlignAxisB=+Y  BaseAlignAxisB=+Z  RotationStandardAxis=+Z  RotationAngle=0  RotationAngleUnits=deg  RotationArbitraryAxis=[0 0 1]  RotationSequenceAxes=FollowerAxes  RotationSequence=XYX  RotationSequenceAngles=[0 0 0]  RotationSequenceAnglesUnits=deg  RotationMatrix=[1 0 0;0 1 0;0 0 1]  Quaternion=[1 0 0 0]  TranslationMethod=Cartesian  TranslationCartesianOffset=[eta_ground beta_ground zeta_ground]  TranslationCartesianOffsetUnits=m  TranslationStandardAxis=+Z  TranslationStandardOffset=0  TranslationStandardOffsetUnits=m  TranslationROffset=0  TranslationROffsetUnits=m  TranslationThetaOffset=0  TranslationThetaOffsetUnits=deg  TranslationZOffset=0  TranslationZOffsetUnits=m
  Conn1 : PMIOPort  Side=Left
  connections:
  Rigid Transform/RConn1 -- Rigid Transform1/LConn1 -- Mounting/RConn1
  Rigid Transform1/RConn1 -- Ground/RConn1
  Rigid Transform/LConn1 -- Conn1/RConn1

== system RedCrane_Merged_control_12032025/Subsystem1 ==
  PS : Gain  Gain=1/1e5
  PS-Simulink Converter2 : nesl_utility/PS-Simulink Converter  PhysicalDomain=network_engine_domain  SubClassName=ps_output  LeftPortType=input  RightPortType=output  PseudoPeriodic=off  Frequencies=[]  VectorFormat=inherit  Unit=inherit  AffineConversion=off
  Pressure Sensor (IL) : fl_lib/Isothermal Liquid/Sensors/Pressure Sensor (IL)  pressure_measure=foundation.enum.pressure_measure.gauge
      settings: InternalSimscapePortConfiguration="{\"Bottom\":[],\"Left\":[{\"id\":\"A\",\"label\":\"A\",\"type\":\"foundation.isothermal_liquid.isothermal_liquid\"}],\"Right\":[{\"id\":\"Pg\",\"label\":\"Pg\",\"type\":\"output\"}],\"Top\":[]}"
  Scope2 : Scope
  Conn1 : PMIOPort  Side=Left
  Ps : Outport
  wires:
  PS-Simulink Converter2/1 -> PS/1
  PS/1 -> Ps/1, Scope2/1
  connections:
  PS-Simulink Converter2/LConn1 -- Pressure Sensor (IL)/RConn1
  Pressure Sensor (IL)/LConn1 -- Conn1/RConn1
